simulink model "closed_loop_model_2019"  (R2019b)
settings: Solver=VariableStepAuto  StartTime=0.0  StopTime=10.0  RelTol=1e-3
undefined symbols (not defined in the file or in its folder): A, B, C, D, K
settings Model: Creator=elina  LastModifiedBy=gebruiker

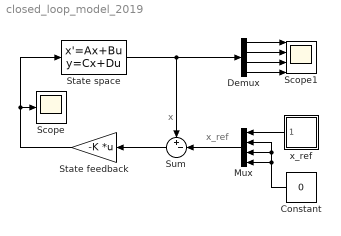
== system closed_loop_model_2019 ==
  note: x
  note: x_ref
  Constant : Constant  Value=0
  Demux : Demux
  Mux : Mux
  Scope : Scope
  Scope1 : Scope  NumInputPorts=4
  State feedback : Gain  Gain=-K  Multiplication=Matrix(K*u)
  State space : StateSpace  A=A  B=B  C=C  D=D  InitialCondition=0
  Sum : Sum  Inputs=+-|
  x_ref : Subsystem
  wires:
  State space/1 -> Demux/1, Sum/1
  Demux/1 -> Scope1/1
  Demux/2 -> Scope1/2
  Demux/3 -> Scope1/3
  Demux/4 -> Scope1/4
  State feedback/1 -> Scope/1, State space/1
  Sum/1 -> State feedback/1
  Mux/1 -> Sum/2
  Constant/1 -> Mux/2, Mux/3, Mux/4
  x_ref/1(Out1) -> Mux/1

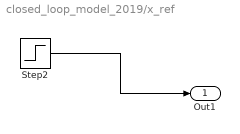
== system closed_loop_model_2019/x_ref ==
  Step2 : Step  SampleTime=0
  Out1 : Outport
  wires:
  Step2/1 -> Out1/1
